simulink model "SRG_Generic_1HpSepExt_13Jan15_mod2"  (Simulink 8.1)
settings: Solver=ode45  StartTime=0.0  StopTime=10  FixedStep=Ts  MaxStep=1e-6  MinStep=1e-7  RelTol=1e-5
values from neighbouring files (symbols this model uses):
  Ts = 1e-06    [WorkSpaceBackup1.mat]
undefined symbols (not defined in the file or in its folder): DiscIntNeverNeededParam, find_system, sigbuilder_block
libraries: powerlib x30, dspsigops x5, simulink_extras x4, simulink x3, powerlib_extras x2, DRlib x1
settings Model: Creator=Rahul  LastModifiedBy=USER
settings DataIOCC: SignalLoggingName=signout
settings OptimizationCC: InitFltsAndDblsToZero=on
settings DebuggingCC: CheckExecutionContextPreStartOutputMsg=on  CheckExecutionContextRuntimeOutputMsg=on  SolverPrmCheckMsg=none  MultiTaskDSMMsg=warning  MultiTaskCondExecSysMsg=none
settings HardwareCC: TargetHWDeviceType=32-bit Generic

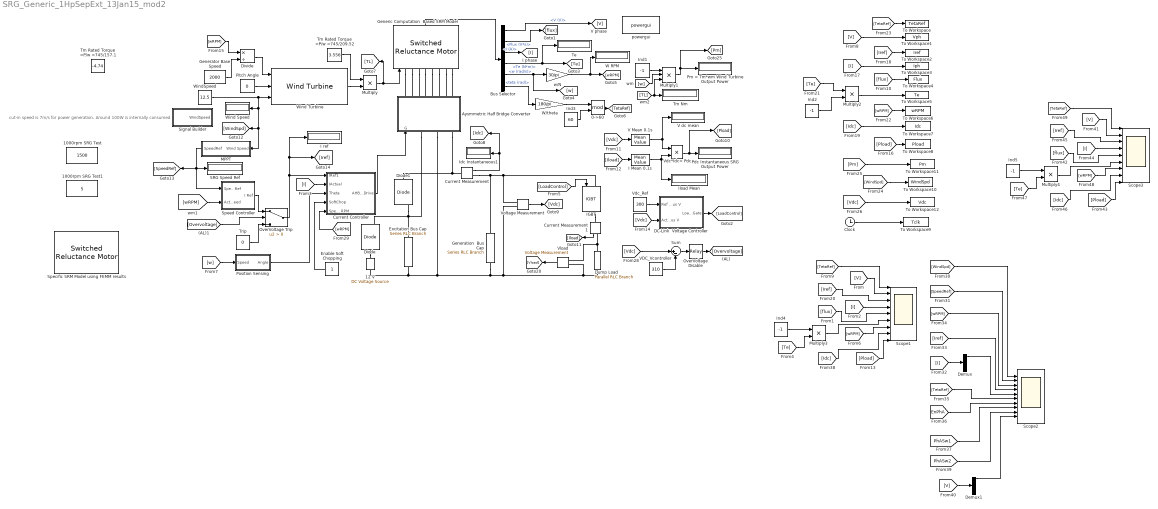
== system SRG_Generic_1HpSepExt_13Jan15_mod2 ==
  note: cut-in speed is 7m/s
      | for power generation.
      | Around 100W is internally consumed
  0->60 : Math  Operator=mod  SampleTime=Ts  SaturateOnIntegerOverflow=on
  1000rpm SRG Test : Constant  Value=1500
  1000rpm SRG Test1 : Constant  Value=5
  12 V : powerlib/Electrical Sources/DC Voltage Source  Amplitude=12  Measurements=None
  Aysmmetric Half Bridge Converter : Subsystem  LoadFcn=find_system(gcs,'FollowLinks', 'on', 'LookUnderMasks', 'all');
  Bus Selector : BusSelector  OutputSignals=V (V),Flux (V*s),I (A),Te (N*m),w (rad/s),teta (rad)
  Clock : Clock
  Current Controller : Subsystem
  Current Measurement : powerlib/Measurements/Current Measurement  PhasorSimulation=off  OutputType=Complex  PSBequivalent=0
  Current Measurement1 : powerlib/Measurements/Current Measurement  PhasorSimulation=off  OutputType=Complex  PSBequivalent=0
  DC-Link  Voltage Controller : Subsystem
  Demux : Demux
  Demux1 : Demux
  Diode : powerlib/Power Electronics/Diode  Ron=0.001  Lon=0  Vf=0.8  IC=0  UseSnubber=off  Rs=10e6  Cs=inf  Measurements=on
  Diode1 : powerlib/Power Electronics/Diode  Ron=0.001  Lon=0  Vf=0.8  IC=0  UseSnubber=off  Rs=10e6  Cs=inf  Measurements=on
  Divide : Product  Inputs=*/
  Dump Load : powerlib/Elements/Parallel RLC Branch  LConnTagsString=a  RConnTagsString=__new0  BranchType=R  Resistance=1  Inductance=1e-3  SetiL0=off  InitialCurrent=0  Capacitance=1e-6  Setx0=off  InitialVoltage=0  Measurements=None
  Enable Soft Chopping : Constant
  Excitation Bus Cap : powerlib/Elements/Series RLC Branch  LConnTagsString=__new0  RConnTagsString=__new0  BranchType=RC  Resistance=0.001  Inductance=1e-3  SetiL0=off  InitialCurrent=0  Capacitance=680e-6  Setx0=on  InitialVoltage=295  Measurements=None
  Generation  Bus Cap : powerlib/Elements/Series RLC Branch  LConnTagsString=__new0  RConnTagsString=__new0  BranchType=RC  Resistance=0.001  Inductance=1e-3  SetiL0=off  InitialCurrent=0  Capacitance=1200e-6  Setx0=on  InitialVoltage=295  Measurements=None
  Generator Base Speed : Constant  Value=2000
  "Generic Computation  Based SRM Model  " : powerlib/Machines/Switched Reluctance Motor  MachineType=8/6  MachineModel=Generic model  StatorResistance=2.15  PlotCurves=off  Inertia=0.004  Friction=0  InitialSpeed=[199 0]  Lq=0.0087  Ld=0.25  Lsat=0.0005  MaximumCurrent=5  MaximumFluxLinkage=0.3  MagnetisationCharacteristic='srm64_60kw.mat'  RotorAngleVector=[0 10 20 30 40 45]  StatorCurrentVector=0:25:450  TsPowergui=0  TsBlock=-1
  I Mean 0.1s : powerlib_extras/Measurements/Mean Value  Period=0.015
  I ref : Display
  IGBT : powerlib/Power Electronics/IGBT  Ron=0.001  Lon=0  Vf=1  Tf=1e-6  Tt=2e-6  IC=0  Rs=1e5  Cs=inf  Measurements=on
  Idc Instantaneous1 : Display
  Iload Mean : Display
  Ind{1..2,4..5} (4 alike) : Constant  Value=-1
  Ind3 : Constant  Value=60
  MPPT : Subsystem
  Multiply{,2..4} (4 alike) : Product  Inputs=**
  Multiply1 : Product  Inputs=***
  OverVoltage Disable : Relay  OnSwitchValue=0  OffSwitchValue=-10  OnOutputValue=0  OffOutputValue=1
  OverVoltage Trip : Switch  Criteria=u2 > Threshold
  Pdc Instantaneous SRG Output Power : Display
  Pitch Angle : Constant  Value=0
  Pm = Tm*wm Wind Turbine Output Power : Display
  Position Sensing : Subsystem
  SRG Speed Ref : Display
  Scope1 : Scope  NumInputPorts=9
      settings: TimeRange=1  YMin=0~-400~0~0~-0.1~0~2000~-5~450  YMax=62~400~5.5~6.5~0.4~5~2005~15~550  SaveName=ScopeData2  MaxDataPoints=1000000
  Scope2 : Scope  NumInputPorts=10
      settings: TimeRange=1  YMin=12~1999~1999~0~0~0~0~0~0~-350  YMax=13~2002~2005~6.5~6.5~62~1.1~1.1~1.1~350  SaveName=ScopeData3  MaxDataPoints=1000000
  Scope3 : Scope  NumInputPorts=9
      settings: TimeRange=1  YMin=0~-400~0~0~-0.1~0~2000~-5~450  YMax=62~400~6.5~6.5~0.4~5~2005~15~550  SaveName=ScopeData5  MaxDataPoints=100000
  Signal Builder : Subsystem  Tag=STV Subsys  LoadFcn=sigbuilder_block('load');  StartFcn=sigbuilder_block('start');  StopFcn=sigbuilder_block('stop');  ClipboardFcn=sigbuilder_block('clipboard');  mask(Sigbuilder block){}
      mask help: Simulink:masks:SigbuilderBlock_MD
      mask init:
      | if ~strcmp(get_param(bdroot(gcbh),'SimulationStatus'),'stopped') tuvar = sigbuilder_block('maskInit'); end
      settings: CopyFcn=sigbuilder_block('copy');  DeleteFcn=sigbuilder_block('delete');  ModelCloseFcn=sigbuilder_block('modelClose');  PreSaveFcn=sigbuilder_block('preSave');  PauseFcn=sigbuilder_block('pause');  ContinueFcn=sigbuilder_block('continue');  NameChangeFcn=sigbuilder_block('namechange');  OpenFcn=sigbuilder_block('open',[0 28.5 1191 582.75 ]);  CloseFcn=sigbuilder_block('close');
      mask Display: plot(0, 0, 100, 100,[2, 2, 32, 32, 2], [68, 8, 8, 68, 68],[32, 2], [38, 38], [32, 19, 2],[53, 60, 44], [32, 17, 17, 2],[16, 16, 31, 31]);txt = getActiveGroup(gcbh);text(2, 100, txt,'verticalAlignment', 'top');
  Specific SRM Model using FEMM results : powerlib/Machines/Switched Reluctance Motor  MachineType=8/6  MachineModel=Specific model  StatorResistance=2.15  PlotCurves=off  Inertia=0.004  Friction=0  InitialSpeed=[199 0]  Lq=0.0087  Ld=0.25  Lsat=0.0005  MaximumCurrent=5  MaximumFluxLinkage=0.3  MagnetisationCharacteristic='SRM86HP1.mat'  RotorAngleVector=[0 1 2 3 4 5 6 7 8 9 10 11 12 13 14 15 16 17 18 19 20 21 22 23 24 25 26 27 28 29 30 31 32 33 34 35 36 37 38 39 40 41 42 43 44 45 46 47 48 49 50 51 52 53 54 55 56 57 58 59 60]  StatorCurrentVector=[0.1 0.2 0.3 0.5 1 1.5 2 2.5 3 3.5 4 4.5 5 5.5 6]  TsPowergui=0  TsBlock=-1
  Speed Controller : Subsystem
  Sum : Sum  Inputs=|+-
  Te : Display
  Tm Nm : Display
  Tm Rated Torque =P/w =745/157.1 : Constant  Value=-4.74
  Tm Rated Torque =P/w =745/209.52 : Constant  Value=3.556
  To Workspace : ToWorkspace  VariableName=TetaRef  SampleTime=-1  SaveFormat=Timeseries
  To Workspace1 : ToWorkspace  VariableName=Vph  SampleTime=-1  SaveFormat=Timeseries
  To Workspace10 : ToWorkspace  VariableName=WindSpd  SampleTime=-1  SaveFormat=Timeseries
  To Workspace11 : ToWorkspace  VariableName=Pm  SampleTime=-1  SaveFormat=Timeseries
  To Workspace12 : ToWorkspace  VariableName=Vdc  SampleTime=-1  SaveFormat=Timeseries
  To Workspace2 : ToWorkspace  VariableName=Iref  SampleTime=-1  SaveFormat=Timeseries
  To Workspace3 : ToWorkspace  VariableName=Iph  SampleTime=-1  SaveFormat=Timeseries
  To Workspace4 : ToWorkspace  VariableName=Flux  SampleTime=-1  SaveFormat=Timeseries
  To Workspace5 : ToWorkspace  VariableName=Te  SampleTime=-1  SaveFormat=Timeseries
  To Workspace6 : ToWorkspace  VariableName=wRPM  SampleTime=-1  SaveFormat=Timeseries
  To Workspace7 : ToWorkspace  VariableName=Idc  SampleTime=-1  SaveFormat=Timeseries
  To Workspace8 : ToWorkspace  VariableName=Pload  SampleTime=-1  SaveFormat=Timeseries
  To Workspace9 : ToWorkspace  VariableName=Tclk  SampleTime=-1  SaveFormat=Timeseries
  Trip : Constant  Value=0
  V Mean 0.1s : powerlib_extras/Measurements/Mean Value  Period=0.015
  V dc mean : Display
  VDC_Vcontroller : Constant  Value=310
  Vdc*Idc= Pdc : Product
  Vdc_Ref : Constant  Value=300
  Vload : powerlib/Measurements/Voltage Measurement  PhasorSimulation=off  OutputType=Complex  PSBequivalent=0
  Voltage Measurement : powerlib/Measurements/Voltage Measurement  PhasorSimulation=off  OutputType=Complex  PSBequivalent=0
  W RPM : Display
  W/theta : Gain  Gain=180/pi
  Wind Speed : Display
  Wind Turbine : DRlib/Wind Generation/Wind Turbine  Pnom=745  Pelec_base=745  wind_base=12.5  P_wind_base=1  speed_nom=1  pitch_angle=0  DisplayTurbChar=off  c1_c6="[0.51763          116          0.4            5           21     0.006795]"  cp_nom=0.48  lambda_nom=8.1
  WindSpeed : Constant  Value=12.5
  powergui : powerlib/powergui  Priority=1  SimulationMode=Discrete  SolverType=Tustin  SampleTime=Ts  frequency=60  SPID=off  DisableSnubberDevices=off  DisableRonSwitches=off  DisableVfSwitches=off  SwTol=0  Interpol=off  DisplayEquations=off  frequencyindice=0  Pbase=100e6  ErrMax=1e-4  Iterations=50  UnitsV=kV  UnitsW=MW  FunctionMessages=off  echomessages=off  HookPort=off  EnableUseOfTLC=off  x0status=blocks  RestoreLinks=warning  ResistiveCurrentMeasurement=off  Frange=[0:2:500]  Ylog=off  Xlog=on  ShowGrid=off  save=off  variable=ZData  ZoomFFT=off  StartTime=0.0  cycles=1  DisplayStyle=1  fundamental=60  FreqAxis=off  MaxFrequency=1000  frequencyindicesteady=1  RmsSteady=1  display=off  Ts=0  methode=off
  w/N : Gain  Gain=30/pi
  wires:
  "Generic Computation  Based SRM Model  "/1 -> Bus Selector/1
  Bus Selector/6 -> W/theta/1  "<teta (rad)>"
  w/N/1 -> [wRPM], W RPM/1
  Ind3/1 -> 0->60/2
  W/theta/1 -> 0->60/1
  Bus Selector/1 -> [V]  "<V (V)>"
  Bus Selector/2 -> [flux]  "<Flux (V*s)>"
  Bus Selector/3 -> [I]  "<I (A)>"
  Bus Selector/4 -> Te/1, [Te]  "<Te (N*m)>"
  Bus Selector/5 -> w/N/1, [w]  "<w (rad/s)>"
  0->60/1 -> [TetaRef]
  Voltage Measurement/1 -> [Vdc]
  Current Measurement/1 -> Idc Instantaneous1/1, [Idc]
  [Iload] -> I Mean 0.1s/1
  Vdc*Idc= Pdc/1 -> Pdc Instantaneous SRG Output Power/1, [Pload]
  Current Measurement1/1 -> [Iload]
  [w] -> Multiply1/2
  Multiply1/1 -> Pm = Tm*wm Wind Turbine Output Power/1, [Pm]
  [Vdc] -> V Mean 0.1s/1
  I Mean 0.1s/1 -> Vdc*Idc= Pdc/2, Iload Mean/1
  Vload/1 -> [Vload]
  V Mean 0.1s/1 -> Vdc*Idc= Pdc/1, V dc mean/1
  [w] -> Position Sensing/1(Speed)
  [TetaRef] -> Scope1/1
  [V] -> Scope1/2
  [Iref] -> Scope1/3
  [I] -> Scope1/4
  [Pload] -> Scope1/9
  [Idc] -> Scope1/8
  [wRPM] -> Scope1/7
  [flux] -> Scope1/5
  [LoadControl] -> IGBT/1
  Vdc_Ref/1 -> DC-Link  Voltage Controller/1(Ref Gen Bus V)
  [Vdc] -> DC-Link  Voltage Controller/2(Actual Gen Bus V)
  DC-Link  Voltage Controller/1(" Load Gate") -> [LoadControl]
  [wRPM] -> Speed Controller/2(ActualSpeed)
  [I] -> Current Controller/2(IActual)
  Current Controller/1(AHB GateDrive) -> Aysmmetric Half Bridge Converter/1(G)
  [wRPM] -> Divide/1
  Generator Base Speed/1 -> Divide/2
  Divide/1 -> Wind Turbine/1
  Pitch Angle/1 -> Wind Turbine/2
  Wind Turbine/1 -> Multiply/2
  [TL] -> Multiply1/3, Tm Nm/1
  Position Sensing/1(Angle) -> Current Controller/3(Theta)
  Enable Soft Chopping/1 -> Current Controller/4(SoftChop)
  [TetaRef] -> To Workspace/1
  [V] -> To Workspace1/1
  [Iref] -> To Workspace2/1
  [I] -> To Workspace3/1
  [Pload] -> To Workspace8/1
  [Idc] -> To Workspace7/1
  [wRPM] -> To Workspace6/1
  [flux] -> To Workspace4/1
  Clock/1 -> To Workspace9/1
  [WindSpd] -> To Workspace10/1
  [Pm] -> To Workspace11/1
  [Vdc] -> To Workspace12/1
  Tm Rated Torque =P/w =745/209.52/1 -> Multiply/1
  Multiply/1 -> "Generic Computation  Based SRM Model  "/1, [TL]
  Trip/1 -> OverVoltage Trip/3
  [Overvoltage] -> OverVoltage Trip/2
  Speed Controller/1(I Ref) -> OverVoltage Trip/1
  OverVoltage Trip/1 -> Current Controller/1(IRef1), I ref/1, [Iref]
  Sum/1 -> OverVoltage Disable/1
  OverVoltage Disable/1 -> [Overvoltage]
  [Vdc] -> Sum/1
  VDC_Vcontroller/1 -> Sum/2
  [wRPM] -> Current Controller/5(Speed RPM)
  Ind1/1 -> Multiply1/1
  [Te] -> Multiply2/1
  Multiply2/1 -> To Workspace5/1
  Ind2/1 -> Multiply2/2
  Multiply3/1 -> Scope1/6
  [Te] -> Multiply3/2
  Ind4/1 -> Multiply3/1
  WindSpeed/1 -> MPPT/1(Wind Speed), [WindSpd], Wind Speed/1, Wind Turbine/3
  MPPT/1(SpeedRef) -> [SpeedRef], SRG Speed Ref/1, Speed Controller/1(SpeedRef)
  [V] -> Demux1/1
  [I] -> Demux/1
  [WindSpd] -> Scope2/1
  [SpeedRef] -> Scope2/2
  [wRPM] -> Scope2/3
  [Iref] -> Scope2/4
  Demux/1 -> Scope2/5
  [TetaRef] -> Scope2/6
  [EnPhA] -> Scope2/7
  [PhASw1] -> Scope2/8
  [PhASw2] -> Scope2/9
  Demux1/1 -> Scope2/10
  [TetaRef] -> Scope3/1
  [V] -> Scope3/2
  [Iref] -> Scope3/3
  [I] -> Scope3/4
  [Pload] -> Scope3/9
  [Idc] -> Scope3/8
  [wRPM] -> Scope3/7
  [flux] -> Scope3/5
  Multiply4/1 -> Scope3/6
  [Te] -> Multiply4/2
  Ind5/1 -> Multiply4/1
  connections:
  "Generic Computation  Based SRM Model  "/LConn1 -- Aysmmetric Half Bridge Converter/RConn1
  "Generic Computation  Based SRM Model  "/LConn2 -- Aysmmetric Half Bridge Converter/RConn2
  "Generic Computation  Based SRM Model  "/LConn3 -- Aysmmetric Half Bridge Converter/RConn3
  "Generic Computation  Based SRM Model  "/LConn4 -- Aysmmetric Half Bridge Converter/RConn4
  "Generic Computation  Based SRM Model  "/LConn5 -- Aysmmetric Half Bridge Converter/RConn5
  "Generic Computation  Based SRM Model  "/LConn6 -- Aysmmetric Half Bridge Converter/RConn6
  Voltage Measurement/LConn2 -- 12 V/LConn1 -- Excitation Bus Cap/RConn1 -- Aysmmetric Half Bridge Converter/LConn2 -- Generation  Bus Cap/RConn1 -- Dump Load/RConn1 -- Vload/LConn2
  Voltage Measurement/LConn1 -- IGBT/LConn1 -- Current Measurement/RConn1 -- Generation  Bus Cap/LConn1
  Diode/LConn1 -- 12 V/RConn1
  Dump Load/LConn1 -- Vload/LConn1 -- Current Measurement1/RConn1
  IGBT/RConn1 -- Current Measurement1/LConn1
  "Generic Computation  Based SRM Model  "/LConn7 -- Aysmmetric Half Bridge Converter/RConn7
  "Generic Computation  Based SRM Model  "/LConn8 -- Aysmmetric Half Bridge Converter/RConn8
  Aysmmetric Half Bridge Converter/LConn3 -- Current Measurement/LConn1 -- Diode1/LConn1
  Aysmmetric Half Bridge Converter/LConn1 -- Diode/RConn1 -- Excitation Bus Cap/LConn1 -- Diode1/RConn1

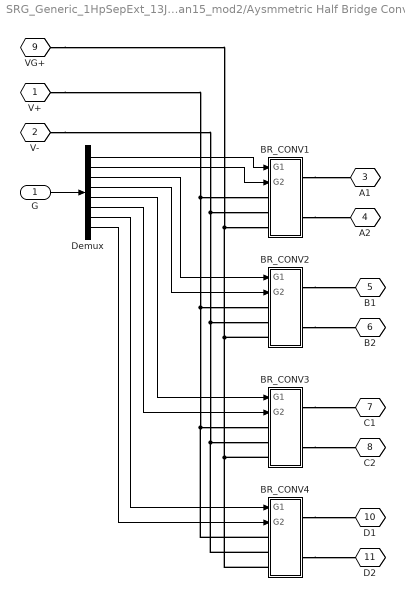
== system SRG_Generic_1HpSepExt_13Jan15_mod2/Aysmmetric Half Bridge Converter ==
  G : Inport
  BR_CONV1 : Subsystem
  BR_CONV2 : Subsystem
  BR_CONV3 : Subsystem
  BR_CONV4 : Subsystem
  Demux : Demux  Outputs=8
  V+ : PMIOPort  Tag=PMCPort  Port=1  Side=Left
  V- : PMIOPort  Tag=PMCPort  Port=2  Side=Left
  A1 : PMIOPort  Tag=PMCPort  Port=3  Side=Right
  A2 : PMIOPort  Tag=PMCPort  Port=4  Side=Right
  B1 : PMIOPort  Tag=PMCPort  Port=5  Side=Right
  B2 : PMIOPort  Tag=PMCPort  Port=6  Side=Right
  C1 : PMIOPort  Tag=PMCPort  Port=7  Side=Right
  C2 : PMIOPort  Tag=PMCPort  Port=8  Side=Right
  VG+ : PMIOPort  Tag=PMCPort  Port=9  Side=Left
  D1 : PMIOPort  Tag=PMCPort  Port=10  Side=Right
  D2 : PMIOPort  Tag=PMCPort  Port=11  Side=Right
  wires:
  G/1 -> Demux/1
  Demux/1 -> BR_CONV1/1(G1)
  Demux/2 -> BR_CONV1/2(G2)
  Demux/3 -> BR_CONV2/1(G1)
  Demux/4 -> BR_CONV2/2(G2)
  Demux/5 -> BR_CONV3/1(G1)
  Demux/6 -> BR_CONV3/2(G2)
  Demux/7 -> BR_CONV4/1(G1)
  Demux/8 -> BR_CONV4/2(G2)
  connections:
  BR_CONV3/RConn2 -- C2/RConn1
  BR_CONV3/RConn1 -- C1/RConn1
  BR_CONV2/RConn2 -- B2/RConn1
  BR_CONV2/RConn1 -- B1/RConn1
  BR_CONV1/RConn2 -- A2/RConn1
  BR_CONV1/RConn1 -- A1/RConn1
  V-/RConn1 -- BR_CONV1/LConn2 -- BR_CONV4/LConn2 -- BR_CONV3/LConn2 -- BR_CONV2/LConn2
  V+/RConn1 -- BR_CONV1/LConn1 -- BR_CONV4/LConn1 -- BR_CONV3/LConn1 -- BR_CONV2/LConn1
  VG+/RConn1 -- BR_CONV1/LConn3 -- BR_CONV4/LConn3 -- BR_CONV3/LConn3 -- BR_CONV2/LConn3
  BR_CONV4/RConn2 -- D2/RConn1
  BR_CONV4/RConn1 -- D1/RConn1

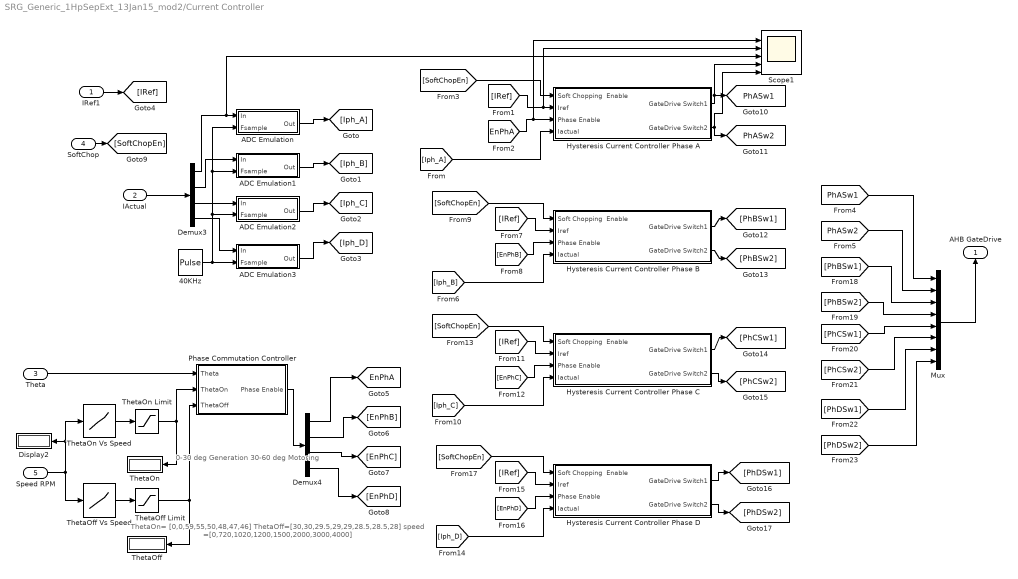
== system SRG_Generic_1HpSepExt_13Jan15_mod2/Current Controller ==
  note: ThetaOn= [0,0,59,55,50,48,47,46]
      | ThetaOff=[30,30,29.5,29,29,28.5,28.5,28]
      | speed =[0,720,1020,1200,1500,2000,3000,4000]
  note: 0-30 deg Generation
      | 30-60 deg Motoring
  IRef1 : Inport
  IActual : Inport  Port=2
  Theta : Inport  Port=3
  SoftChop : Inport  Port=4
  Speed RPM : Inport  Port=5
  40KHz : DiscretePulseGenerator  PulseType=Time based  Period=0.25e-4  PulseWidth=10
  ADC Emulation : Subsystem
  ADC Emulation1 : Subsystem
  ADC Emulation2 : Subsystem
  ADC Emulation3 : Subsystem
  Demux3 : Demux
  Demux4 : Demux
  Display2 : Display
  Hysteresis Current Controller Phase A : Subsystem
  Hysteresis Current Controller Phase B : Subsystem
  Hysteresis Current Controller Phase C : Subsystem
  Hysteresis Current Controller Phase D : Subsystem
  Mux : Mux  Inputs=8
  Phase Commutation Controller : Subsystem
  Scope1 : Scope  NumInputPorts=6
      settings: YMin=0~0~-0.1~-0.1~0~0  YMax=65~1.1~6~6~1.1~1.1  SaveName=ScopeData4  MaxDataPoints=500000
  ThetaOff : Display
  ThetaOff Limit : Saturate  UpperLimit=60  LowerLimit=0
  ThetaOff Vs Speed : Lookup_n-D  NumberOfTableDimensions=1  BreakpointsForDimension1=[0,720,1020,1200,1500,2000,3000,4000]  Table=[30,30,29.5,29,29,28.5,28.5,28]  TableMin=0  TableMax=60  InterpMethod=Cubic spline  ExtrapMethod=Cubic spline  RndMeth=Simplest  InputSameDT=on
  ThetaOn : Display
  ThetaOn Limit : Saturate  UpperLimit=60  LowerLimit=0
  ThetaOn Vs Speed : Lookup_n-D  NumberOfTableDimensions=1  BreakpointsForDimension1=[0,720,1020,1200,1500,2000,3000,4000]  Table=[0,0,59,55,50,48,47,46]  TableMin=0  TableMax=60  InterpMethod=Cubic spline  ExtrapMethod=Cubic spline  RndMeth=Simplest  InputSameDT=on
  AHB GateDrive : Outport
  tag scope: EnPhA=global, PhASw1=global, PhASw2=global
  wires:
  IActual/1 -> Demux3/1
  Mux/1 -> AHB GateDrive/1
  IRef1/1 -> [IRef]
  Theta/1 -> Phase Commutation Controller/1(Theta)
  Phase Commutation Controller/1(Phase Enable) -> Demux4/1
  Demux4/1 -> [EnPhA]
  Demux4/2 -> [EnPhB]
  Demux4/3 -> [EnPhC]
  Demux4/4 -> [EnPhD]
  SoftChop/1 -> [SoftChopEn]
  [PhASw1] -> Mux/1
  [PhASw2] -> Mux/2
  [SoftChopEn] -> Hysteresis Current Controller Phase A/1(Soft Chopping  Enable)
  [IRef] -> Scope1/3, Hysteresis Current Controller Phase A/2(Iref)
  [EnPhA] -> Scope1/2, Hysteresis Current Controller Phase A/3(Phase Enable)
  [Iph_A] -> Hysteresis Current Controller Phase A/4(Iactual)
  Hysteresis Current Controller Phase A/2(GateDrive Switch2) -> Scope1/6, [PhASw2]
  [SoftChopEn] -> Hysteresis Current Controller Phase B/1(Soft Chopping  Enable)
  [IRef] -> Hysteresis Current Controller Phase B/2(Iref)
  [EnPhB] -> Hysteresis Current Controller Phase B/3(Phase Enable)
  [Iph_B] -> Hysteresis Current Controller Phase B/4(Iactual)
  Hysteresis Current Controller Phase B/1(GateDrive Switch1) -> [PhBSw1]
  Hysteresis Current Controller Phase B/2(GateDrive Switch2) -> [PhBSw2]
  [SoftChopEn] -> Hysteresis Current Controller Phase C/1(Soft Chopping  Enable)
  [IRef] -> Hysteresis Current Controller Phase C/2(Iref)
  [EnPhC] -> Hysteresis Current Controller Phase C/3(Phase Enable)
  [Iph_C] -> Hysteresis Current Controller Phase C/4(Iactual)
  Hysteresis Current Controller Phase C/1(GateDrive Switch1) -> [PhCSw1]
  Hysteresis Current Controller Phase C/2(GateDrive Switch2) -> [PhCSw2]
  [SoftChopEn] -> Hysteresis Current Controller Phase D/1(Soft Chopping  Enable)
  [IRef] -> Hysteresis Current Controller Phase D/2(Iref)
  [EnPhD] -> Hysteresis Current Controller Phase D/3(Phase Enable)
  [Iph_D] -> Hysteresis Current Controller Phase D/4(Iactual)
  Hysteresis Current Controller Phase D/1(GateDrive Switch1) -> [PhDSw1]
  Hysteresis Current Controller Phase D/2(GateDrive Switch2) -> [PhDSw2]
  [PhBSw1] -> Mux/3
  [PhBSw2] -> Mux/4
  [PhCSw1] -> Mux/5
  [PhCSw2] -> Mux/6
  [PhDSw1] -> Mux/7
  [PhDSw2] -> Mux/8
  Demux3/1 -> Scope1/4, ADC Emulation/1(In)
  Demux3/2 -> ADC Emulation1/1(In)
  Demux3/3 -> ADC Emulation2/1(In)
  Demux3/4 -> ADC Emulation3/1(In)
  40KHz/1 -> ADC Emulation2/2(Fsample), ADC Emulation/2(Fsample), ADC Emulation1/2(Fsample), ADC Emulation3/2(Fsample)
  Speed RPM/1 -> ThetaOn Vs Speed/1, Display2/1, ThetaOff Vs Speed/1
  ThetaOn Vs Speed/1 -> ThetaOn Limit/1
  ThetaOn Limit/1 -> ThetaOn/1, Phase Commutation Controller/2("ThetaOn ")
  ThetaOff Vs Speed/1 -> ThetaOff Limit/1
  ThetaOff Limit/1 -> ThetaOff/1, Phase Commutation Controller/3(ThetaOff)
  ADC Emulation/1(Out) -> [Iph_A]
  ADC Emulation1/1(Out) -> [Iph_B]
  ADC Emulation2/1(Out) -> [Iph_C]
  ADC Emulation3/1(Out) -> [Iph_D]
  Hysteresis Current Controller Phase A/1(GateDrive Switch1) -> Scope1/5, [PhASw1]

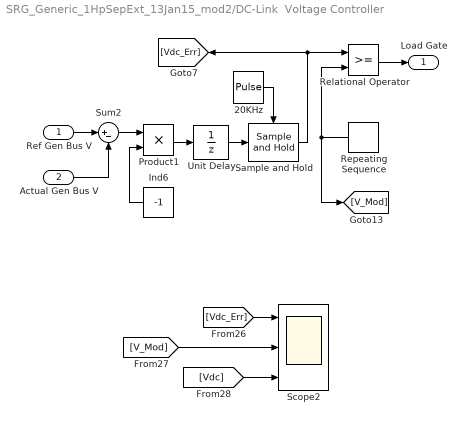
== system SRG_Generic_1HpSepExt_13Jan15_mod2/DC-Link  Voltage Controller ==
  Ref Gen Bus V : Inport
  Actual Gen Bus V : Inport  Port=2
  20KHz : DiscretePulseGenerator  PulseType=Time based  Period=0.5e-4  PulseWidth=10
  Ind6 : Constant  Value=-1
  Product1 : Product
  Relational Operator : RelationalOperator  OutDataTypeStr=boolean
  Repeating Sequence : simulink/Sources/Repeating Sequence  rep_seq_t=[0 0.25e-4 0.5e-4]  rep_seq_y=[0 1 0]
  Sample and Hold : dspsigops/Sample and Hold  trig=Rising edge  initCond=0  latchinput=off
  Scope2 : Scope  NumInputPorts=3
      settings: TimeRange=0.1400000000000001  YMin=-5~-2~0  YMax=5~2~300  MaxDataPoints=100000
  Sum2 : Sum  Inputs=|+-
  Unit Delay : UnitDelay  SampleTime=-1
  " Load Gate" : Outport
  wires:
  Ref Gen Bus V/1 -> Sum2/1
  Actual Gen Bus V/1 -> Sum2/2
  [V_Mod] -> Scope2/2
  [Vdc] -> Scope2/3
  20KHz/1 -> Sample and Hold/Trigger
  Repeating Sequence/1 -> Relational Operator/2, [V_Mod]
  [Vdc_Err] -> Scope2/1
  Ind6/1 -> Product1/2
  Product1/1 -> Unit Delay/1
  Unit Delay/1 -> Sample and Hold/1
  Sample and Hold/1 -> Relational Operator/1, [Vdc_Err]
  Sum2/1 -> Product1/1
  Relational Operator/1 -> " Load Gate"/1

== system SRG_Generic_1HpSepExt_13Jan15_mod2/MPPT ==
  Wind Speed : Inport
  Correction factor : Constant
  Gear : Constant  Value=5.0469
  LAMDA : Constant  Value=8.1
  Turbine Radius : Constant  Value=2.439
  W_opt calc. for MPPT : Product  Inputs=*****/
  rad/s to rpm : Constant  Value=9.549
  SpeedRef : Outport
  wires:
  Gear/1 -> W_opt calc. for MPPT/3
  LAMDA/1 -> W_opt calc. for MPPT/2
  Turbine Radius/1 -> W_opt calc. for MPPT/6
  rad/s to rpm/1 -> W_opt calc. for MPPT/4
  Wind Speed/1 -> W_opt calc. for MPPT/1
  W_opt calc. for MPPT/1 -> SpeedRef/1
  Correction factor/1 -> W_opt calc. for MPPT/5

== system SRG_Generic_1HpSepExt_13Jan15_mod2/Position Sensing ==
  Speed : Inport
  Constant2 : Constant  Value=60
  Discrete-Time Integrator2 : DiscreteIntegrator  InitialCondition=[0 -15 -30 -45]  SampleTime=Ts  ICPrevOutput=DiscIntNeverNeededParam  ICPrevScaledInput=DiscIntNeverNeededParam
  Elect. Angle 0-60 (deg) : Display
  Gain1 : Gain  Gain=180/pi  SaturateOnIntegerOverflow=on  OutDataTypeStr=Inherit: Same as input  ParamDataTypeStr=Inherit: Same as input
  Math Function2 : Math  Operator=mod  SaturateOnIntegerOverflow=on
  Mech. Angle [0 to 360] +[360*rotations] (deg) : Display
  Speed (deg/s) : Display
  Angle : Outport
  wires:
  Constant2/1 -> Math Function2/2
  Discrete-Time Integrator2/1 -> Math Function2/1, Mech. Angle [0 to 360] +[360*rotations] (deg)/1
  Speed/1 -> Gain1/1
  Math Function2/1 -> Angle/1, Elect. Angle 0-60 (deg)/1
  Gain1/1 -> Speed (deg/s)/1, Discrete-Time Integrator2/1

== system SRG_Generic_1HpSepExt_13Jan15_mod2/Signal Builder ==
  Demux : Demux  Tag=STV Demux  Outputs=1
  FromWs : FromWorkspace  Tag=STV FromWs  VariableName=tuvar  SampleTime=0  SigBuilderData=DataTag0  VnvData=DataTag1
      SigBuilderData=|
      | common.afterFinalStr = 'Extrapolate'
      | common.sampleTime = 0
      | dataSet.timeRange = [0 10]
      | dataSet.name = 'Group 1'
      | sbobj.Groups.Name = 'Group 1'
      | sbobj.Groups.Signals.Name = 'WindSpeed'
      | sbobj.Groups.Signals.XData = [0 3.33 5 6.66 6.66 10]
      | sbobj.Groups.Signals.YData = [8.6 8.6 13.8 13.8 12.5 12.5]
  WindSpeed : Outport  Tag=STV Outport
  wires:
  FromWs/1 -> Demux/1
  Demux/1 -> WindSpeed/1

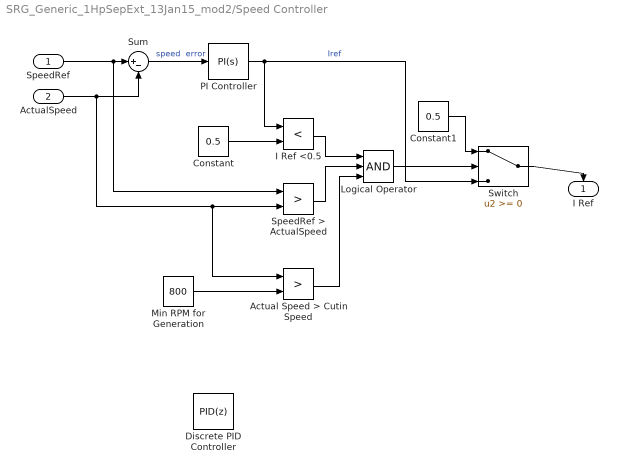
== system SRG_Generic_1HpSepExt_13Jan15_mod2/Speed Controller ==
  SpeedRef : Inport
  ActualSpeed : Inport  Port=2
  Actual Speed > Cutin Speed : RelationalOperator  Operator=>  OutDataTypeStr=boolean
  Constant : Constant  Value=0.5
  Constant1 : Constant  Value=0.5
  Discrete PID Controller : simulink/Continuous/PID Controller  Controller=PID  TimeDomain=Discrete-time  SampleTime=1  IntegratorMethod=Forward Euler  FilterMethod=Forward Euler  Form=Parallel  P=1  I=1  D=0  N=100  InitialConditionSource=internal  InitialConditionForIntegrator=0  InitialConditionForFilter=0  ExternalReset=none  LimitOutput=off  UpperSaturationLimit=inf  LowerSaturationLimit=-inf  LinearizeAsGain=off  AntiWindupMode=none  Kb=1  TrackingMode=off  Kt=1  PParamMin=[]  PParamMax=[]  IParamMin=[]  IParamMax=[]  DParamMin=[]  DParamMax=[]  NParamMin=[]  NParamMax=[]  KbParamMin=[]  KbParamMax=[]  KtParamMin=[]  KtParamMax=[]  POutMin=[]  POutMax=[]  IOutMin=[]  IOutMax=[]  DOutMin=[]  DOutMax=[]  NOutMin=[]  NOutMax=[]  KbOutMin=[]  KbOutMax=[]  KtOutMin=[]  KtOutMax=[]  IntegratorOutMin=[]  IntegratorOutMax=[]  FilterOutMin=[]  FilterOutMax=[]  SumOutMin=[]  SumOutMax=[]  SumI1OutMin=[]  SumI1OutMax=[]  SumI2OutMin=[]  SumI2OutMax=[]  SumI3OutMin=[]  SumI3OutMax=[]  SumDOutMin=[]  SumDOutMax=[]  SaturationOutMin=[]  SaturationOutMax=[]  IntegratorContinuousStateAttributes=''  IntegratorStateMustResolveToSignalObject=off  IntegratorRTWStateStorageClass=Auto  FilterContinuousStateAttributes=''  FilterStateMustResolveToSignalObject=off  FilterRTWStateStorageClass=Auto
  I Ref <0.5 : RelationalOperator  Operator=<  OutDataTypeStr=boolean
  Logical Operator : Logic  Inputs=3  AllPortsSameDT=off  OutDataTypeStr=boolean
  Min RPM for Generation : Constant  Value=800
  PI Controller : simulink/Continuous/PID Controller  Controller=PI  TimeDomain=Continuous-time  SampleTime=Ts  IntegratorMethod=Trapezoidal  FilterMethod=Forward Euler  Form=Parallel  P=-1  I=-5  D=0  N=100  InitialConditionSource=internal  InitialConditionForIntegrator=0  InitialConditionForFilter=0  ExternalReset=none  ZeroCross=off  LimitOutput=on  UpperSaturationLimit=5.5  LowerSaturationLimit=0  LinearizeAsGain=off  AntiWindupMode=clamping  Kb=1  TrackingMode=off  Kt=1  PParamMin=[]  PParamMax=[]  IParamMin=[]  IParamMax=[]  DParamMin=[]  DParamMax=[]  NParamMin=[]  NParamMax=[]  KbParamMin=[]  KbParamMax=[]  KtParamMin=[]  KtParamMax=[]  POutMin=[]  POutMax=[]  IOutMin=[]  IOutMax=[]  DOutMin=[]  DOutMax=[]  NOutMin=[]  NOutMax=[]  KbOutMin=[]  KbOutMax=[]  KtOutMin=[]  KtOutMax=[]  IntegratorOutMin=[]  IntegratorOutMax=[]  FilterOutMin=[]  FilterOutMax=[]  SumOutMin=[]  SumOutMax=[]  SumI1OutMin=[]  SumI1OutMax=[]  SumI2OutMin=[]  SumI2OutMax=[]  SumI3OutMin=[]  SumI3OutMax=[]  SumDOutMin=[]  SumDOutMax=[]  SaturationOutMin=[]  SaturationOutMax=[]  IntegratorContinuousStateAttributes=''  IntegratorStateMustResolveToSignalObject=off  IntegratorRTWStateStorageClass=Auto  FilterContinuousStateAttributes=''  FilterStateMustResolveToSignalObject=off  FilterRTWStateStorageClass=Auto
  SpeedRef > ActualSpeed : RelationalOperator  Operator=>  OutDataTypeStr=boolean
  Sum : Sum  Inputs=|+-
  Switch : Switch
  I Ref : Outport
  wires:
  ActualSpeed/1 -> Actual Speed > Cutin Speed/1, SpeedRef > ActualSpeed/2, Sum/2
  Sum/1 -> PI Controller/1  "speed  error"
  PI Controller/1 -> I Ref <0.5/1, Switch/3  "Iref"
  SpeedRef/1 -> SpeedRef > ActualSpeed/1, Sum/1
  Constant/1 -> I Ref <0.5/2
  I Ref <0.5/1 -> Logical Operator/1
  SpeedRef > ActualSpeed/1 -> Logical Operator/2
  Logical Operator/1 -> Switch/2
  Constant1/1 -> Switch/1
  Min RPM for Generation/1 -> Actual Speed > Cutin Speed/2
  Actual Speed > Cutin Speed/1 -> Logical Operator/3
  Switch/1 -> I Ref/1

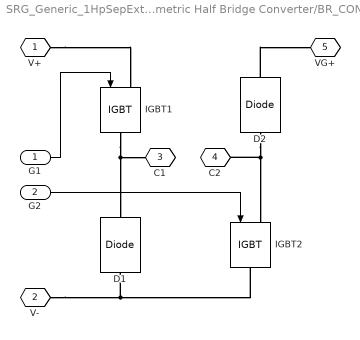
== system SRG_Generic_1HpSepExt_13Jan15_mod2/Aysmmetric Half Bridge Converter/BR_CONV1 ==
  G1 : Inport
  G2 : Inport  Port=2
  D1 : powerlib/Power Electronics/Diode  Ron=1e-3  Lon=0  Vf=0.8  IC=0  UseSnubber=off  Rs=10000  Cs=inf  Measurements=off
  D2 : powerlib/Power Electronics/Diode  Ron=1e-3  Lon=0  Vf=0.8  IC=0  UseSnubber=off  Rs=10000  Cs=inf  Measurements=off
  IGBT1 : powerlib/Power Electronics/IGBT  Ron=1e-3  Lon=0  Vf=1  Tf=0  Tt=0  IC=0  Rs=2000  Cs=0.1e-6  Measurements=off
  IGBT2 : powerlib/Power Electronics/IGBT  Ron=1e-3  Lon=0  Vf=1  Tf=0  Tt=0  IC=0  Rs=2000  Cs=0.1e-6  Measurements=off
  V+ : PMIOPort  Tag=PMCPort  Port=1  Side=Left
  V- : PMIOPort  Tag=PMCPort  Port=2  Side=Left
  C1 : PMIOPort  Tag=PMCPort  Port=3  Side=Right
  C2 : PMIOPort  Tag=PMCPort  Port=4  Side=Right
  VG+ : PMIOPort  Tag=PMCPort  Port=5  Side=Left
  wires:
  G1/1 -> IGBT1/1
  G2/1 -> IGBT2/1
  connections:
  D1/LConn1 -- V-/RConn1 -- IGBT2/RConn1
  D2/LConn1 -- IGBT2/LConn1 -- C2/RConn1
  IGBT1/RConn1 -- D1/RConn1 -- C1/RConn1
  V+/RConn1 -- IGBT1/LConn1
  D2/RConn1 -- VG+/RConn1

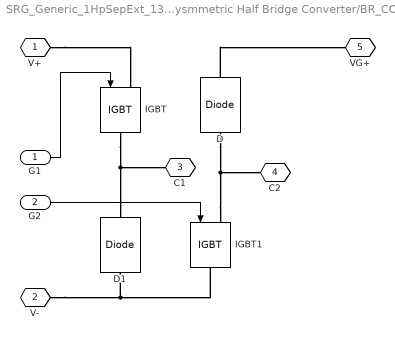
== system SRG_Generic_1HpSepExt_13Jan15_mod2/Aysmmetric Half Bridge Converter/BR_CONV2 ==
  G1 : Inport
  G2 : Inport  Port=2
  D : powerlib/Power Electronics/Diode  Ron=1e-3  Lon=0  Vf=0.8  IC=0  UseSnubber=off  Rs=10000  Cs=inf  Measurements=off
  D1 : powerlib/Power Electronics/Diode  Ron=1e-3  Lon=0  Vf=0.8  IC=0  UseSnubber=off  Rs=10000  Cs=inf  Measurements=off
  IGBT : powerlib/Power Electronics/IGBT  Ron=1e-3  Lon=0  Vf=1  Tf=0  Tt=0  IC=0  Rs=2000  Cs=0.1e-6  Measurements=off
  IGBT1 : powerlib/Power Electronics/IGBT  Ron=1e-3  Lon=0  Vf=1  Tf=0  Tt=0  IC=0  Rs=2000  Cs=0.1e-6  Measurements=off
  V+ : PMIOPort  Tag=PMCPort  Port=1  Side=Left
  V- : PMIOPort  Tag=PMCPort  Port=2  Side=Left
  C1 : PMIOPort  Tag=PMCPort  Port=3  Side=Right
  C2 : PMIOPort  Tag=PMCPort  Port=4  Side=Right
  VG+ : PMIOPort  Tag=PMCPort  Port=5  Side=Left
  wires:
  G1/1 -> IGBT/1
  G2/1 -> IGBT1/1
  connections:
  D1/LConn1 -- V-/RConn1 -- IGBT1/RConn1
  IGBT1/LConn1 -- D/LConn1 -- C2/RConn1
  D1/RConn1 -- IGBT/RConn1 -- C1/RConn1
  V+/RConn1 -- IGBT/LConn1
  D/RConn1 -- VG+/RConn1

== system SRG_Generic_1HpSepExt_13Jan15_mod2/Aysmmetric Half Bridge Converter/BR_CONV3 ==
  G1 : Inport
  G2 : Inport  Port=2
  D : powerlib/Power Electronics/Diode  Ron=1e-3  Lon=0  Vf=0.8  IC=0  UseSnubber=off  Rs=10000  Cs=inf  Measurements=off
  D1 : powerlib/Power Electronics/Diode  Ron=1e-3  Lon=0  Vf=0.8  IC=0  UseSnubber=off  Rs=10000  Cs=inf  Measurements=off
  IGBT : powerlib/Power Electronics/IGBT  Ron=1e-3  Lon=0  Vf=1  Tf=0  Tt=0  IC=0  Rs=2000  Cs=0.1e-6  Measurements=off
  IGBT1 : powerlib/Power Electronics/IGBT  Ron=1e-3  Lon=0  Vf=1  Tf=0  Tt=0  IC=0  Rs=2000  Cs=0.1e-6  Measurements=off
  V+ : PMIOPort  Tag=PMCPort  Port=1  Side=Left
  V- : PMIOPort  Tag=PMCPort  Port=2  Side=Left
  C1 : PMIOPort  Tag=PMCPort  Port=3  Side=Right
  C2 : PMIOPort  Tag=PMCPort  Port=4  Side=Right
  VG+ : PMIOPort  Tag=PMCPort  Port=5  Side=Left
  wires:
  G1/1 -> IGBT/1
  G2/1 -> IGBT1/1
  connections:
  D1/LConn1 -- V-/RConn1 -- IGBT1/RConn1
  IGBT1/LConn1 -- D/LConn1 -- C2/RConn1
  D1/RConn1 -- IGBT/RConn1 -- C1/RConn1
  V+/RConn1 -- IGBT/LConn1
  D/RConn1 -- VG+/RConn1

== system SRG_Generic_1HpSepExt_13Jan15_mod2/Aysmmetric Half Bridge Converter/BR_CONV4 ==
  G1 : Inport
  G2 : Inport  Port=2
  D : powerlib/Power Electronics/Diode  Ron=1e-3  Lon=0  Vf=0.8  IC=0  UseSnubber=off  Rs=10000  Cs=inf  Measurements=off
  D1 : powerlib/Power Electronics/Diode  Ron=1e-3  Lon=0  Vf=0.8  IC=0  UseSnubber=off  Rs=10000  Cs=inf  Measurements=off
  IGBT : powerlib/Power Electronics/IGBT  Ron=1e-3  Lon=0  Vf=1  Tf=0  Tt=0  IC=0  Rs=2000  Cs=0.1e-6  Measurements=off
  IGBT1 : powerlib/Power Electronics/IGBT  Ron=1e-3  Lon=0  Vf=1  Tf=0  Tt=0  IC=0  Rs=2000  Cs=0.1e-6  Measurements=off
  V+ : PMIOPort  Tag=PMCPort  Port=1  Side=Left
  V- : PMIOPort  Tag=PMCPort  Port=2  Side=Left
  C1 : PMIOPort  Tag=PMCPort  Port=3  Side=Right
  C2 : PMIOPort  Tag=PMCPort  Port=4  Side=Right
  VG+ : PMIOPort  Tag=PMCPort  Port=5  Side=Left
  wires:
  G1/1 -> IGBT/1
  G2/1 -> IGBT1/1
  connections:
  D1/LConn1 -- V-/RConn1 -- IGBT1/RConn1
  IGBT1/LConn1 -- D/LConn1 -- C2/RConn1
  D1/RConn1 -- IGBT/RConn1 -- C1/RConn1
  V+/RConn1 -- IGBT/LConn1
  D/RConn1 -- VG+/RConn1

== system SRG_Generic_1HpSepExt_13Jan15_mod2/Current Controller/ADC Emulation ==
  In : Inport
  Fsample : Inport  Port=2
  Sample and Hold : dspsigops/Sample and Hold  trig=Rising edge  initCond=0  latchinput=off
  Out : Outport
  wires:
  Fsample/1 -> Sample and Hold/Trigger
  In/1 -> Sample and Hold/1
  Sample and Hold/1 -> Out/1

== system SRG_Generic_1HpSepExt_13Jan15_mod2/Current Controller/ADC Emulation1 ==
  In : Inport
  Fsample : Inport  Port=2
  Sample and Hold : dspsigops/Sample and Hold  trig=Rising edge  initCond=0  latchinput=off
  Out : Outport
  wires:
  Fsample/1 -> Sample and Hold/Trigger
  In/1 -> Sample and Hold/1
  Sample and Hold/1 -> Out/1

== system SRG_Generic_1HpSepExt_13Jan15_mod2/Current Controller/ADC Emulation2 ==
  In : Inport
  Fsample : Inport  Port=2
  Sample and Hold : dspsigops/Sample and Hold  trig=Rising edge  initCond=0  latchinput=off
  Out : Outport
  wires:
  Fsample/1 -> Sample and Hold/Trigger
  In/1 -> Sample and Hold/1
  Sample and Hold/1 -> Out/1

== system SRG_Generic_1HpSepExt_13Jan15_mod2/Current Controller/ADC Emulation3 ==
  In : Inport
  Fsample : Inport  Port=2
  Sample and Hold : dspsigops/Sample and Hold  trig=Rising edge  initCond=0  latchinput=off
  Out : Outport
  wires:
  Fsample/1 -> Sample and Hold/Trigger
  In/1 -> Sample and Hold/1
  Sample and Hold/1 -> Out/1

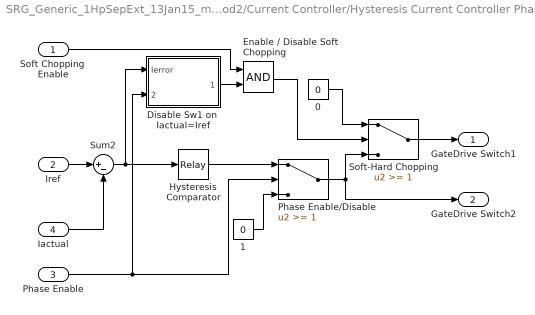
== system SRG_Generic_1HpSepExt_13Jan15_mod2/Current Controller/Hysteresis Current Controller Phase A ==
  Soft Chopping  Enable : Inport
  Iref : Inport  Port=2
  Phase Enable : Inport  Port=3
  Iactual : Inport  Port=4
  0 : Constant  Value=0
  1 : Constant  Value=0
  Disable Sw1 on  Iactual=Iref : Subsystem
  Enable / Disable Soft Chopping : Logic  AllPortsSameDT=off  OutDataTypeStr=boolean
  Hysteresis Comparator : Relay  OnSwitchValue=0.01  OffSwitchValue=-0.01
  "Phase Enable/Disable " : Switch  Threshold=1
  Soft-Hard Chopping : Switch  Threshold=1
  Sum2 : Sum  Inputs=|+-
  GateDrive Switch1 : Outport
  GateDrive Switch2 : Outport  Port=2
  wires:
  Iref/1 -> Sum2/1
  Iactual/1 -> Sum2/2
  Sum2/1 -> Hysteresis Comparator/1, Disable Sw1 on  Iactual=Iref/1(Ierror)
  0/1 -> Soft-Hard Chopping/1
  Disable Sw1 on  Iactual=Iref/1(SwitchDisable) -> Enable / Disable Soft Chopping/2
  Enable / Disable Soft Chopping/1 -> Soft-Hard Chopping/2
  Soft-Hard Chopping/1 -> GateDrive Switch1/1
  Soft Chopping  Enable/1 -> Enable / Disable Soft Chopping/1
  Phase Enable/1 -> Disable Sw1 on  Iactual=Iref/2(Ph_Enable), "Phase Enable/Disable "/2
  "Phase Enable/Disable "/1 -> GateDrive Switch2/1, Soft-Hard Chopping/3
  Hysteresis Comparator/1 -> "Phase Enable/Disable "/1
  1/1 -> "Phase Enable/Disable "/3

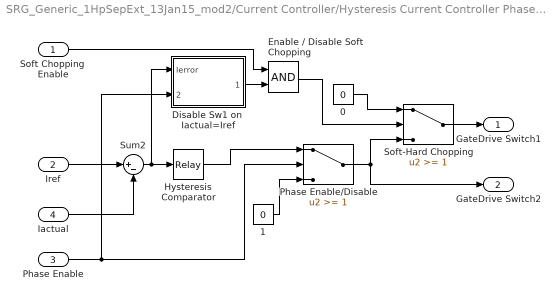
== system SRG_Generic_1HpSepExt_13Jan15_mod2/Current Controller/Hysteresis Current Controller Phase B ==
  Soft Chopping  Enable : Inport
  Iref : Inport  Port=2
  Phase Enable : Inport  Port=3
  Iactual : Inport  Port=4
  0 : Constant  Value=0
  1 : Constant  Value=0
  Disable Sw1 on  Iactual=Iref : Subsystem
  Enable / Disable Soft Chopping : Logic  AllPortsSameDT=off  OutDataTypeStr=boolean
  Hysteresis Comparator : Relay  OnSwitchValue=0.01  OffSwitchValue=-0.01
  "Phase Enable/Disable " : Switch  Threshold=1
  Soft-Hard Chopping : Switch  Threshold=1
  Sum2 : Sum  Inputs=|+-
  GateDrive Switch1 : Outport
  GateDrive Switch2 : Outport  Port=2
  wires:
  Iref/1 -> Sum2/1
  Iactual/1 -> Sum2/2
  Sum2/1 -> Hysteresis Comparator/1, Disable Sw1 on  Iactual=Iref/1(Ierror)
  0/1 -> Soft-Hard Chopping/1
  Disable Sw1 on  Iactual=Iref/1(SwitchDisable) -> Enable / Disable Soft Chopping/2
  Enable / Disable Soft Chopping/1 -> Soft-Hard Chopping/2
  Soft-Hard Chopping/1 -> GateDrive Switch1/1
  Soft Chopping  Enable/1 -> Enable / Disable Soft Chopping/1
  Phase Enable/1 -> Disable Sw1 on  Iactual=Iref/2(Ph_Enable), "Phase Enable/Disable "/2
  "Phase Enable/Disable "/1 -> GateDrive Switch2/1, Soft-Hard Chopping/3
  Hysteresis Comparator/1 -> "Phase Enable/Disable "/1
  1/1 -> "Phase Enable/Disable "/3

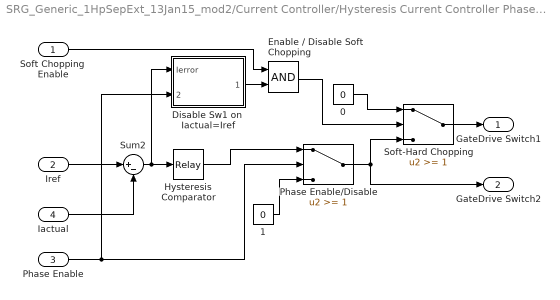
== system SRG_Generic_1HpSepExt_13Jan15_mod2/Current Controller/Hysteresis Current Controller Phase C ==
  Soft Chopping  Enable : Inport
  Iref : Inport  Port=2
  Phase Enable : Inport  Port=3
  Iactual : Inport  Port=4
  0 : Constant  Value=0
  1 : Constant  Value=0
  Disable Sw1 on  Iactual=Iref : Subsystem
  Enable / Disable Soft Chopping : Logic  AllPortsSameDT=off  OutDataTypeStr=boolean
  Hysteresis Comparator : Relay  OnSwitchValue=0.01  OffSwitchValue=-0.01
  "Phase Enable/Disable " : Switch  Threshold=1
  Soft-Hard Chopping : Switch  Threshold=1
  Sum2 : Sum  Inputs=|+-
  GateDrive Switch1 : Outport
  GateDrive Switch2 : Outport  Port=2
  wires:
  Iref/1 -> Sum2/1
  Iactual/1 -> Sum2/2
  Sum2/1 -> Hysteresis Comparator/1, Disable Sw1 on  Iactual=Iref/1(Ierror)
  0/1 -> Soft-Hard Chopping/1
  Disable Sw1 on  Iactual=Iref/1(SwitchDisable) -> Enable / Disable Soft Chopping/2
  Enable / Disable Soft Chopping/1 -> Soft-Hard Chopping/2
  Soft-Hard Chopping/1 -> GateDrive Switch1/1
  Soft Chopping  Enable/1 -> Enable / Disable Soft Chopping/1
  Phase Enable/1 -> Disable Sw1 on  Iactual=Iref/2(Ph_Enable), "Phase Enable/Disable "/2
  "Phase Enable/Disable "/1 -> GateDrive Switch2/1, Soft-Hard Chopping/3
  Hysteresis Comparator/1 -> "Phase Enable/Disable "/1
  1/1 -> "Phase Enable/Disable "/3

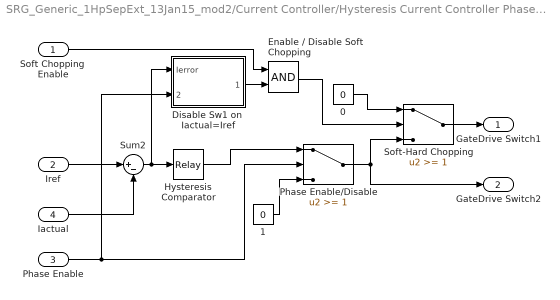
== system SRG_Generic_1HpSepExt_13Jan15_mod2/Current Controller/Hysteresis Current Controller Phase D ==
  Soft Chopping  Enable : Inport
  Iref : Inport  Port=2
  Phase Enable : Inport  Port=3
  Iactual : Inport  Port=4
  0 : Constant  Value=0
  1 : Constant  Value=0
  Disable Sw1 on  Iactual=Iref : Subsystem
  Enable / Disable Soft Chopping : Logic  AllPortsSameDT=off  OutDataTypeStr=boolean
  Hysteresis Comparator : Relay  OnSwitchValue=0.01  OffSwitchValue=-0.01
  "Phase Enable/Disable " : Switch  Threshold=1
  Soft-Hard Chopping : Switch  Threshold=1
  Sum2 : Sum  Inputs=|+-
  GateDrive Switch1 : Outport
  GateDrive Switch2 : Outport  Port=2
  wires:
  Iref/1 -> Sum2/1
  Iactual/1 -> Sum2/2
  Sum2/1 -> Hysteresis Comparator/1, Disable Sw1 on  Iactual=Iref/1(Ierror)
  0/1 -> Soft-Hard Chopping/1
  Disable Sw1 on  Iactual=Iref/1(SwitchDisable) -> Enable / Disable Soft Chopping/2
  Enable / Disable Soft Chopping/1 -> Soft-Hard Chopping/2
  Soft-Hard Chopping/1 -> GateDrive Switch1/1
  Soft Chopping  Enable/1 -> Enable / Disable Soft Chopping/1
  Phase Enable/1 -> Disable Sw1 on  Iactual=Iref/2(Ph_Enable), "Phase Enable/Disable "/2
  "Phase Enable/Disable "/1 -> GateDrive Switch2/1, Soft-Hard Chopping/3
  Hysteresis Comparator/1 -> "Phase Enable/Disable "/1
  1/1 -> "Phase Enable/Disable "/3

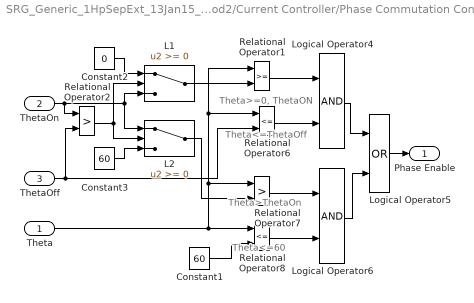
== system SRG_Generic_1HpSepExt_13Jan15_mod2/Current Controller/Phase Commutation Controller ==
  note: Theta<=60
  note: Theta>ThetaOn
  note: Theta<=ThetaOff
  note: Theta>=0, ThetaON
  Theta : Inport
  "ThetaOn " : Inport  Port=2
  ThetaOff : Inport  Port=3
  Constant1 : Constant  Value=60
  Constant2 : Constant  Value=0
  Constant3 : Constant  Value=60
  L1 : Switch
  L2 : Switch
  Logical Operator4 : Logic  AllPortsSameDT=off
  Logical Operator5 : Logic  Operator=OR  AllPortsSameDT=off
  Logical Operator6 : Logic  AllPortsSameDT=off
  Relational Operator1 : RelationalOperator
  Relational Operator2 : RelationalOperator  Operator=>
  Relational Operator6 : RelationalOperator  Operator=<=
  Relational Operator7 : RelationalOperator  Operator=>
  Relational Operator8 : RelationalOperator  Operator=<=
  Phase Enable : Outport
  wires:
  Theta/1 -> Relational Operator7/1, Relational Operator1/1, Relational Operator6/1, Relational Operator8/1
  Relational Operator7/1 -> Logical Operator6/1
  ThetaOff/1 -> Relational Operator2/2, Relational Operator6/2
  L1/1 -> Relational Operator1/2
  Logical Operator5/1 -> Phase Enable/1
  "ThetaOn "/1 -> Relational Operator2/1, L2/1, L1/3
  Relational Operator6/1 -> Logical Operator4/2
  Logical Operator4/1 -> Logical Operator5/1
  Relational Operator1/1 -> Logical Operator4/1
  L2/1 -> Relational Operator7/2
  Logical Operator6/1 -> Logical Operator5/2
  Constant1/1 -> Relational Operator8/2
  Relational Operator8/1 -> Logical Operator6/2
  Relational Operator2/1 -> L2/2, L1/2
  Constant2/1 -> L1/1
  Constant3/1 -> L2/3

== system SRG_Generic_1HpSepExt_13Jan15_mod2/Current Controller/Hysteresis Current Controller Phase A/Disable Sw1 on  Iactual=Iref ==
  Ierror : Inport
  Ph_Enable : Inport  Port=2
  Constant : Constant  Value=0.1
  Constant1 : Constant  Value=0
  Disable  Upper SW on Iref=Iactual : simulink_extras/Flip Flops/S-R Flip-Flop  initial_condition=0
  Ierror~0 Iref=Iactual : RelationalOperator  Operator=<=  OutDataTypeStr=boolean
  "Phase Inactive " : RelationalOperator  Operator=<=  OutDataTypeStr=boolean
  Terminator : Terminator
  SwitchDisable : Outport
  wires:
  Constant/1 -> Ierror~0 Iref=Iactual/2
  Ierror~0 Iref=Iactual/1 -> Disable  Upper SW on Iref=Iactual/1
  Disable  Upper SW on Iref=Iactual/2 -> Terminator/1
  Disable  Upper SW on Iref=Iactual/1 -> SwitchDisable/1
  Constant1/1 -> "Phase Inactive "/2
  Ph_Enable/1 -> "Phase Inactive "/1
  "Phase Inactive "/1 -> Disable  Upper SW on Iref=Iactual/2
  Ierror/1 -> Ierror~0 Iref=Iactual/1

== system SRG_Generic_1HpSepExt_13Jan15_mod2/Current Controller/Hysteresis Current Controller Phase B/Disable Sw1 on  Iactual=Iref ==
  Ierror : Inport
  Ph_Enable : Inport  Port=2
  Constant : Constant  Value=0.1
  Constant1 : Constant  Value=0
  Disable  Upper SW on Iref=Iactual : simulink_extras/Flip Flops/S-R Flip-Flop  initial_condition=0
  Ierror~0 Iref=Iactual : RelationalOperator  Operator=<=  OutDataTypeStr=boolean
  "Phase Inactive " : RelationalOperator  Operator=<=  OutDataTypeStr=boolean
  Terminator : Terminator
  SwitchDisable : Outport
  wires:
  Constant/1 -> Ierror~0 Iref=Iactual/2
  Ierror~0 Iref=Iactual/1 -> Disable  Upper SW on Iref=Iactual/1
  Disable  Upper SW on Iref=Iactual/2 -> Terminator/1
  Disable  Upper SW on Iref=Iactual/1 -> SwitchDisable/1
  Constant1/1 -> "Phase Inactive "/2
  Ph_Enable/1 -> "Phase Inactive "/1
  "Phase Inactive "/1 -> Disable  Upper SW on Iref=Iactual/2
  Ierror/1 -> Ierror~0 Iref=Iactual/1

== system SRG_Generic_1HpSepExt_13Jan15_mod2/Current Controller/Hysteresis Current Controller Phase C/Disable Sw1 on  Iactual=Iref ==
  Ierror : Inport
  Ph_Enable : Inport  Port=2
  Constant : Constant  Value=0.1
  Constant1 : Constant  Value=0
  Disable  Upper SW on Iref=Iactual : simulink_extras/Flip Flops/S-R Flip-Flop  initial_condition=0
  Ierror~0 Iref=Iactual : RelationalOperator  Operator=<=  OutDataTypeStr=boolean
  "Phase Inactive " : RelationalOperator  Operator=<=  OutDataTypeStr=boolean
  Terminator : Terminator
  SwitchDisable : Outport
  wires:
  Constant/1 -> Ierror~0 Iref=Iactual/2
  Ierror~0 Iref=Iactual/1 -> Disable  Upper SW on Iref=Iactual/1
  Disable  Upper SW on Iref=Iactual/2 -> Terminator/1
  Disable  Upper SW on Iref=Iactual/1 -> SwitchDisable/1
  Constant1/1 -> "Phase Inactive "/2
  Ph_Enable/1 -> "Phase Inactive "/1
  "Phase Inactive "/1 -> Disable  Upper SW on Iref=Iactual/2
  Ierror/1 -> Ierror~0 Iref=Iactual/1

== system SRG_Generic_1HpSepExt_13Jan15_mod2/Current Controller/Hysteresis Current Controller Phase D/Disable Sw1 on  Iactual=Iref ==
  Ierror : Inport
  Ph_Enable : Inport  Port=2
  Constant : Constant  Value=0.1
  Constant1 : Constant  Value=0
  Disable  Upper SW on Iref=Iactual : simulink_extras/Flip Flops/S-R Flip-Flop  initial_condition=0
  Ierror~0 Iref=Iactual : RelationalOperator  Operator=<=  OutDataTypeStr=boolean
  "Phase Inactive " : RelationalOperator  Operator=<=  OutDataTypeStr=boolean
  Terminator : Terminator
  SwitchDisable : Outport
  wires:
  Constant/1 -> Ierror~0 Iref=Iactual/2
  Ierror~0 Iref=Iactual/1 -> Disable  Upper SW on Iref=Iactual/1
  Disable  Upper SW on Iref=Iactual/2 -> Terminator/1
  Disable  Upper SW on Iref=Iactual/1 -> SwitchDisable/1
  Constant1/1 -> "Phase Inactive "/2
  Ph_Enable/1 -> "Phase Inactive "/1
  "Phase Inactive "/1 -> Disable  Upper SW on Iref=Iactual/2
  Ierror/1 -> Ierror~0 Iref=Iactual/1
